simulink model "IGBT24V_200A"  (Simulink 8.6)
settings: Solver=ode23tb  StartTime=0.0  StopTime=0.06  MaxStep=1e-6  MinStep=1e-7  RelTol=1e-4
libraries: powerlib x21, powerlib_extras x3, simulink x1
settings Model: Creator=Administrator  LastModifiedBy=wuhaoyu
settings DebuggingCC: FcnCallInpInsideContextMsg=UseLocalSettings

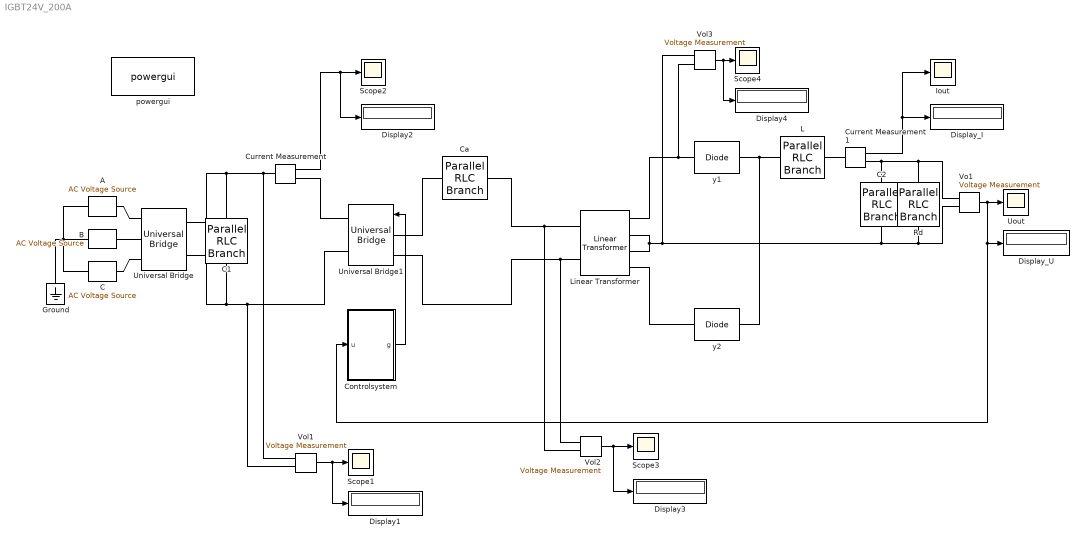
== system IGBT24V_200A ==
  A : powerlib/Electrical Sources/AC Voltage Source  Amplitude=227*sqrt(2)  Phase=0  Frequency=60  SampleTime=50e-6  Measurements=Voltage  BusType=swing  Pref=10e3  Qref=0  Qmin=-inf  Qmax=+inf
  B : powerlib/Electrical Sources/AC Voltage Source  Amplitude=227*sqrt(2)  Phase=-120  Frequency=60  SampleTime=50e-6  Measurements=Voltage  BusType=swing  Pref=10e3  Qref=0  Qmin=-inf  Qmax=+inf
  C : powerlib/Electrical Sources/AC Voltage Source  Amplitude=227*sqrt(2)  Phase=120  Frequency=60  SampleTime=50e-6  Measurements=Voltage  BusType=swing  Pref=10e3  Qref=0  Qmin=-inf  Qmax=+inf
  C1 : powerlib/Elements/Parallel RLC Branch  LConnTagsString=a  RConnTagsString=__new0  BranchType=C  Resistance=1  Inductance=1e-3  SetiL0=off  InitialCurrent=0  Capacitance=3e-6  Setx0=off  InitialVoltage=0  Measurements=None
  C2 : powerlib/Elements/Parallel RLC Branch  LConnTagsString=a  RConnTagsString=__new0  BranchType=C  Resistance=1  Inductance=1e-3  SetiL0=off  InitialCurrent=0  Capacitance=1000e-6  Setx0=off  InitialVoltage=0  Measurements=None
  Ca : powerlib/Elements/Parallel RLC Branch  LConnTagsString=a  RConnTagsString=__new0  BranchType=C  Resistance=1  Inductance=15E-6  SetiL0=off  InitialCurrent=0  Capacitance=30e-6  Setx0=off  InitialVoltage=0  Measurements=Branch current
  Controlsystem : Subsystem
  Current Measurement : powerlib/Measurements/Current Measurement  PhasorSimulation=off  OutputType=Complex  PSBequivalent=0
  Current Measurement1 : powerlib/Measurements/Current Measurement  PhasorSimulation=off  OutputType=Complex  PSBequivalent=0
  Display{1..4} (4 alike) : Display
  Display_I : Display
  Display_U : Display
  Ground : powerlib/Elements/Ground  LConnTagsString=a
  Iout : Scope
  L : powerlib/Elements/Parallel RLC Branch  LConnTagsString=a  RConnTagsString=__new0  BranchType=L  Resistance=1  Inductance=2e-3  SetiL0=off  InitialCurrent=0  Capacitance=1e-6  Setx0=off  InitialVoltage=0  Measurements=Branch current
  Linear Transformer : powerlib/Elements/Linear Transformer  UNITS=SI  NominalPower=[5.6e+5 20000]  winding1=[800 0.00175 1e-005]  winding2=[40 3.5714e-005 1.421e-013]  ThreeWindings=on  winding3=[40 3.5714e-005 1.421e-013]  RmLm=[4.375 0.028]  Measurements=Winding voltages  DataType=on
  Rd : powerlib/Elements/Parallel RLC Branch  LConnTagsString=a  RConnTagsString=__new0  BranchType=R  Resistance=0.5  Inductance=1e-3  SetiL0=off  InitialCurrent=0  Capacitance=1e-6  Setx0=off  InitialVoltage=0  Measurements=Branch voltage and current
  Scope{1..4} (4 alike) : Scope
  Universal Bridge : powerlib/Power Electronics/Universal Bridge  Arms=3  SnubberResistance=1e5  SnubberCapacitance=1e-6  Device=Diodes  Ron=1e-3  Lon=0  ForwardVoltages="[  0  0  ]"  ForwardVoltage=0  GTOparameters=[ 10e-6 , 20e-6 ]  IGBTparameters=[ 1e-6 , 2e-6 ]  Measurements=None  Measurements_2=None  converterType=Rectifier
  Universal Bridge1 : powerlib/Power Electronics/Universal Bridge  Arms=2  SnubberResistance=1e5  SnubberCapacitance=1e-6  Device=IGBT / Diodes  Ron=1e-3  Lon=0  ForwardVoltages="[  0  0  ]"  ForwardVoltage=0  GTOparameters=[ 10e-6 , 20e-6 ]  IGBTparameters=[ 1e-6 , 2e-6 ]  Measurements=All voltages and currents  Measurements_2=None  converterType=Rectifier
  Uout : Scope
  Vo1 : powerlib/Measurements/Voltage Measurement  PhasorSimulation=off  OutputType=Complex  PSBequivalent=0
  Vol1 : powerlib/Measurements/Voltage Measurement  PhasorSimulation=off  OutputType=Complex  PSBequivalent=0
  Vol2 : powerlib/Measurements/Voltage Measurement  PhasorSimulation=off  OutputType=Complex  PSBequivalent=0
  Vol3 : powerlib/Measurements/Voltage Measurement  PhasorSimulation=off  OutputType=Complex  PSBequivalent=0
  powergui : powerlib/powergui  SimulationMode=Discrete  SolverType=Tustin/Backward Euler (TBE)  SampleTime=1e-6  frequency=60  SPID=off  DisableSnubberDevices=off  DisableRonSwitches=off  DisableVfSwitches=off  SwTol=0  DisplayEquations=off  Interpol=off  ExternalGateDelay=off  methode=off  Ts=0  FunctionMessages=off  echomessages=off  HookPort=off  EnableUseOfTLC=off  x0status=blocks  frequencyindice=60  Pbase=100e6  ErrMax=1e-4  Iterations=50  UnitsV=kV  UnitsW=MW  buscounter=0  RestoreLinks=warning  ResistiveCurrentMeasurement=off  Frange=[0:2:500]  Ylog=off  Xlog=on  ShowGrid=off  save=off  variable=ZData  structure=0  ZoomFFT=on  StartTime=0.0  cycles=1  DisplayStyle=1  fundamental=60  FreqAxis=off  MaxFrequency=1000  frequencyindicesteady=1  RmsSteady=1  display=off
  y1 : powerlib/Power Electronics/Diode  Ron=0.001  Lon=0  Vf=0.8  IC=0  UseSnubber=off  Rs=500  Cs=0.047e-6  Measurements=off
  y2 : powerlib/Power Electronics/Diode  Ron=0.001  Lon=0  Vf=0.8  IC=0  UseSnubber=off  Rs=500  Cs=0.047e-6  Measurements=off
  wires:
  Controlsystem/1(g) -> Universal Bridge1/1
  Vol1/1 -> Scope1/1, Display1/1
  Current Measurement1/1 -> Iout/1, Display_I/1
  Current Measurement/1 -> Scope2/1, Display2/1
  Vol2/1 -> Scope3/1, Display3/1
  Vo1/1 -> Uout/1, Display_U/1, Controlsystem/1(u)
  Vol3/1 -> Scope4/1, Display4/1
  connections:
  C/LConn1 -- B/LConn1 -- A/LConn1 -- Ground/LConn1
  Current Measurement/LConn1 -- Vol1/LConn1 -- Universal Bridge/RConn1 -- C1/LConn1
  Universal Bridge1/RConn2 -- Vol1/LConn2 -- Universal Bridge/RConn2 -- C1/RConn1
  Ca/LConn1 -- Universal Bridge1/LConn1
  Universal Bridge1/LConn2 -- Linear Transformer/LConn2 -- Vol2/LConn1
  Current Measurement/RConn1 -- Universal Bridge1/RConn1
  Ca/RConn1 -- Linear Transformer/LConn1 -- Vol2/LConn2
  Linear Transformer/RConn4 -- y2/LConn1
  y1/LConn1 -- Linear Transformer/RConn1 -- Vol3/LConn2
  Current Measurement1/RConn1 -- C2/LConn1 -- Vo1/LConn1 -- Rd/LConn1
  y1/RConn1 -- L/LConn1 -- y2/RConn1
  L/RConn1 -- Current Measurement1/LConn1
  Linear Transformer/RConn3 -- Linear Transformer/RConn2 -- Vol3/LConn1 -- C2/RConn1 -- Vo1/LConn2 -- Rd/RConn1
  Universal Bridge/LConn1 -- A/RConn1
  Universal Bridge/LConn2 -- B/RConn1
  Universal Bridge/LConn3 -- C/RConn1

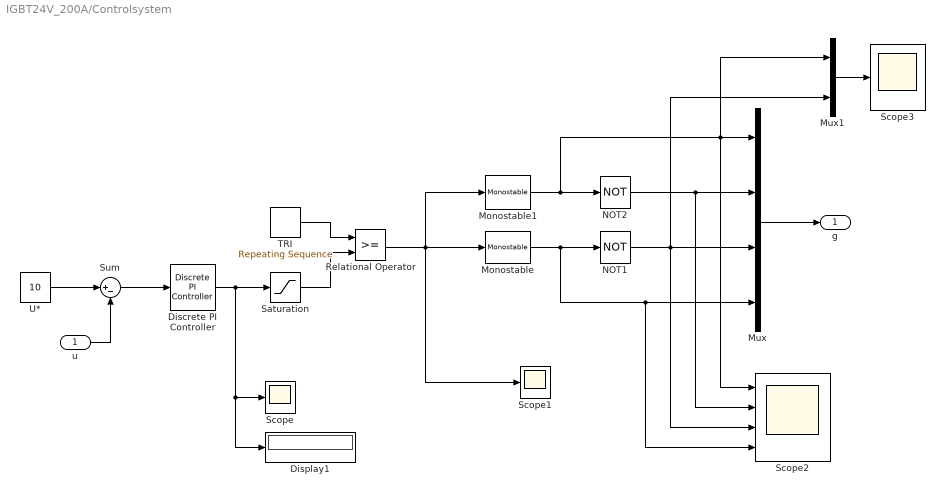
== system IGBT24V_200A/Controlsystem ==
  u : Inport
  Discrete PI Controller : powerlib_extras/Discrete  Control Blocks/Discrete PI Controller  Kp=0.5  Ki=0.8  Par_Limits=[1e6 -1e6]  Init=0  Ts=50e-6
  Display1 : Display
  Monostable : powerlib_extras/Control  Blocks/Monostable  EdgeDetect=Falling  t_mono=1/(2*20000)  ic=0
  Monostable1 : powerlib_extras/Control  Blocks/Monostable  EdgeDetect=Rising  t_mono=1/(2*20000)  ic=0
  Mux : Mux
  Mux1 : Mux  Inputs=2
  NOT1 : Logic  Operator=NOT  AllPortsSameDT=off  OutDataTypeStr=boolean
  NOT2 : Logic  Operator=NOT  AllPortsSameDT=off  OutDataTypeStr=boolean
  Relational Operator : RelationalOperator  OutDataTypeStr=boolean
  Saturation : Saturate  UpperLimit=0.85  LowerLimit=0.01
  Scope : Scope
  Scope1 : Scope
  Scope2 : Scope  NumInputPorts=4
  Scope3 : Scope
  Sum : Sum  Inputs=|+-
  TRI : simulink/Sources/Repeating Sequence  rep_seq_t=[0 1/(4*20000) 1/(2*20000) 3/(4*20000) 1/20000]  rep_seq_y=[0 1 0 -1 0]
  U* : Constant  Value=10
  g : Outport
  wires:
  Sum/1 -> Discrete PI Controller/1
  U*/1 -> Sum/1
  TRI/1 -> Relational Operator/1
  Saturation/1 -> Relational Operator/2
  Relational Operator/1 -> Monostable/1, Scope1/1, Monostable1/1
  Monostable1/1 -> NOT2/1, Mux/1, Scope2/1, Mux1/1
  Monostable/1 -> NOT1/1, Mux/4, Scope2/4
  NOT2/1 -> Mux/2, Scope2/2
  NOT1/1 -> Mux/3, Scope2/3, Mux1/2
  u/1 -> Sum/2
  Discrete PI Controller/1 -> Saturation/1, Scope/1, Display1/1
  Mux/1 -> g/1
  Mux1/1 -> Scope3/1
